simulink model "Lab2_DCmach"  (R2021b)
settings: Solver=ode45  StartTime=0.0  StopTime=10.0  MaxStep=1e-3  RelTol=1e-6  EnableMultiTasking=on
values from neighbouring files (symbols this model uses):
  B = 0.004    [Lab2_DCmachControl.m]
  J = 0.054    [Lab2_DCmachControl.m]
  La = .01985    (= 0.01985)    [Lab2_DCmachControl.m]
  lambda = K_lambda*ifeild    (= 1.266)    [Lab2_DCmachControl.m]
  Ra = 1.9    [Lab2_DCmachControl.m]
  TL_step = 0    [Lab2_DCmachControl.m]
  TL_steptime1 = 0    [Lab2_DCmachControl.m]
  TL_steptime2 = 0    [Lab2_DCmachControl.m]
  vT_step = 180    [Lab2_DCmachControl.m]
  vT_steptime = 0.1    [Lab2_DCmachControl.m]
settings Model: Creator=andlinds  LastModifiedBy=emmag
settings SolverCC: AlgebraicLoopSolver=TrustRegion
settings DataIOCC: LimitDataPoints=on  SaveFormat=Array  SignalLoggingSaveFormat=ModelDataLogs  ReturnWorkspaceOutputs=off
settings OptimizationCC: ExpressionDepthLimit=2147483647  InitFltsAndDblsToZero=on  LifeSpan=inf
settings DebuggingCC: UnderspecifiedInitializationDetection=Classic  MergeDetectMultiDrivingBlocksExec=none  FcnCallInpInsideContextMsg=warning  StateNameClashWarn=warning  SFUnexpectedBacktrackingDiag=warning  SFNoUnconditionalDefaultTransitionDiag=warning  SFExecutionAtInitializationDiag=none  SFMachineParentedDataDiag=warning  ArithmeticOperatorsInVariantConditions=warning
settings HardwareCC: ProdBitPerPointer=32  ProdBitPerSizeT=32  ProdBitPerPtrDiffT=32  ProdLargestAtomicFloat=None  ProdIntDivRoundTo=Undefined  ProdEndianess=Unspecified  ProdWordSize=32  ProdHWDeviceType=32-bit Generic
settings ModelReferenceCC: PropagateSignalLabelsOutOfModel=off
settings SFSimCC: SimUseLocalCustomCode=off  CustomCodeUndefinedFunction=UseInterfaceOnly
settings RTWCC: RTWUseLocalCustomCode=off
settings CodeAppCC: StateflowObjectComments=on
settings GRTTargetCC: TargetLangStandard=C89/C90 (ANSI)  CombineOutputUpdateFcns=off  GRTInterface=on
settings ConfigComp: CovMetricSettings=dw  CovSaveCumulativeToWorkspaceVar=on  CovSaveSingleToWorkspaceVar=on  CovExternalEMLEnable=off

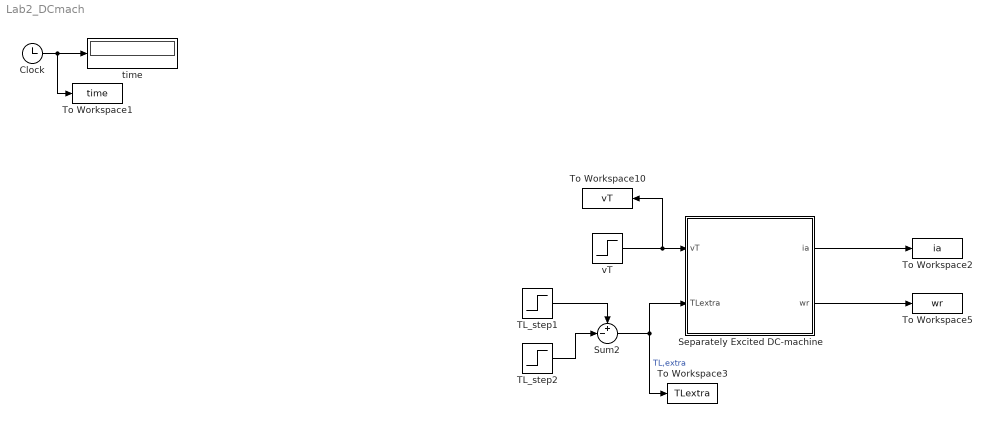
== system Lab2_DCmach ==
  Clock : Clock
  Separately Excited DC-machine : Subsystem
  Sum2 : Sum  Inputs=+-|
  TL_step1 : Step  Time=TL_steptime1  After=TL_step  SampleTime=0
  TL_step2 : Step  Time=TL_steptime2  After=TL_step*2  SampleTime=0
  To Workspace1 : ToWorkspace  VariableName=time  SampleTime=-1
  To Workspace10 : ToWorkspace  VariableName=vT  SampleTime=-1
  To Workspace2 : ToWorkspace  VariableName=ia  SampleTime=-1
  To Workspace3 : ToWorkspace  VariableName=TLextra  SampleTime=-1
  To Workspace5 : ToWorkspace  VariableName=wr  SampleTime=-1
  time : Display
  vT : Step  Time=vT_steptime  After=vT_step  SampleTime=0
  wires:
  Clock/1 -> time/1, To Workspace1/1
  vT/1 -> Separately Excited DC-machine/1(vT), To Workspace10/1
  Separately Excited DC-machine/1(ia) -> To Workspace2/1
  Separately Excited DC-machine/2(wr) -> To Workspace5/1
  TL_step1/1 -> Sum2/1
  TL_step2/1 -> Sum2/2
  Sum2/1 -> Separately Excited DC-machine/2(TLextra), To Workspace3/1  "TL,extra"

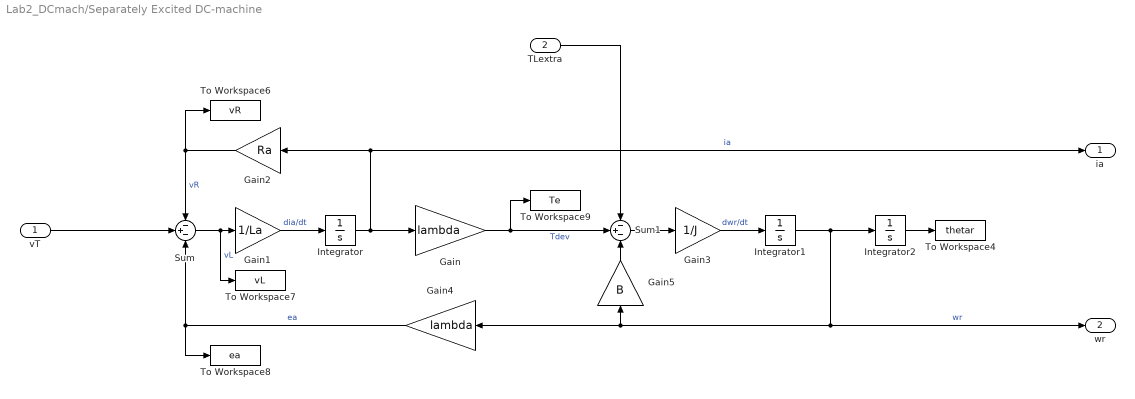
== system Lab2_DCmach/Separately Excited DC-machine ==
  vT : Inport
  TLextra : Inport  Port=2
  Gain : Gain  Gain=lambda
  Gain1 : Gain  Gain=1/La
  Gain2 : Gain  Gain=Ra
  Gain3 : Gain  Gain=1/J
  Gain4 : Gain  Gain=lambda
  Gain5 : Gain  Gain=B
  Integrator : Integrator
  Integrator1 : Integrator
  Integrator2 : Integrator
  Sum : Sum  Inputs=-+-
  Sum1 : Sum  Inputs=-+-
  To Workspace4 : ToWorkspace  VariableName=thetar  SampleTime=-1
  To Workspace6 : ToWorkspace  VariableName=vR  SampleTime=-1
  To Workspace7 : ToWorkspace  VariableName=vL  SampleTime=-1
  To Workspace8 : ToWorkspace  VariableName=ea  SampleTime=-1
  To Workspace9 : ToWorkspace  VariableName=Te  SampleTime=-1
  ia : Outport  VectorParamsAs1DForOutWhenUnconnected=off
  wr : Outport  Port=2  VectorParamsAs1DForOutWhenUnconnected=off
  wires:
  Integrator/1 -> Gain/1, ia/1, Gain2/1  "ia"
  Gain1/1 -> Integrator/1  "dia/dt"
  Gain/1 -> Sum1/2, To Workspace9/1  "Tdev"
  Gain3/1 -> Integrator1/1  "dwr/dt"
  Integrator2/1 -> To Workspace4/1
  Gain5/1 -> Sum1/3
  Sum1/1 -> Gain3/1
  Integrator1/1 -> Integrator2/1, wr/1, Gain4/1, Gain5/1  "wr"
  Gain4/1 -> Sum/3, To Workspace8/1  "ea"
  Sum/1 -> Gain1/1, To Workspace7/1  "vL"
  Gain2/1 -> Sum/1, To Workspace6/1  "vR"
  vT/1 -> Sum/2
  TLextra/1 -> Sum1/1
